simulink model "UAV_sync_unknown"  (R2018a)
settings: Solver=ode23tb  StartTime=0.0  StopTime=40
values from neighbouring files (symbols this model uses):
  Bm = [zeros(6); eye(6)]    [UAV_sync_unknown.m]    (also in UAV_sync_unknown_Node1.m = [zeros(6,6);ones(6,6)]; UAV_sync_unknown_Node2.m)
  C_rho = 1.225    [SC42120_UAV_Preconditions.m]
  D0 = [M0 0 0 0 0 0 ... (first row only)    [SC42120_UAV_Preconditions.m]
  Derivative_gain_phi = 50    [SC42120_UAV_Preconditions.m]
  Derivative_gain_psi = 50    [SC42120_UAV_Preconditions.m]
  Derivative_gain_theta = 50    [SC42120_UAV_Preconditions.m]
  Derivative_gain_x = 50    [SC42120_UAV_Preconditions.m]
  Derivative_gain_y = 50    [SC42120_UAV_Preconditions.m]
  Derivative_gain_z = 50    [SC42120_UAV_Preconditions.m]
  G = 9.80665    [SC42120_UAV_Preconditions.m]
  g0 = [0;0;-M0*G;0;0;0]    [SC42120_UAV_Preconditions.m]
  I0 = [0.02 0 -0.01 ... (first row only)    [SC42120_UAV_Preconditions.m]
  InitWind = [0;0;0]    [SC42120_UAV_Preconditions.m]
  Kp = diag(P)    [SC42120_UAV_Preconditions.m]
  Kv = diag(V)    [SC42120_UAV_Preconditions.m]
  M0 = 10    [SC42120_UAV_Preconditions.m]
  Pm = lyap(Am',-100*eye(12))    [UAV_sync_unknown_Node1.m]    (also in UAV_sync_unknown_Node2.m = lyap(Am',100*eye(12)))
  Proportional_phi = 50    [SC42120_UAV_Preconditions.m]
  Proportional_psi = 50    [SC42120_UAV_Preconditions.m]
  Proportional_theta = 50    [SC42120_UAV_Preconditions.m]
  Proportional_x = 50    [SC42120_UAV_Preconditions.m]
  Proportional_y = 50    [SC42120_UAV_Preconditions.m]
  Proportional_z = 50    [SC42120_UAV_Preconditions.m]
  S1 = eye(6)*1    [UAV_sync_unknown.m]    (also in UAV_sync_unknown_Node1.m = eye(6))
  S2 = eye(6)*1    [UAV_sync_unknown.m]    (also in UAV_sync_unknown_Node2.m)
undefined symbols (not defined in the file or in its folder): Aero, APlane, Bxl, C, Ctr, deg, DiscIntNeverNeededParam, F, Guid, Init, Light, MIL, Path, rad, s, Trim, Utility
libraries: aerolibconvert2 x37, simulink x15, dspsigops x7, shared6dof x6, aerolibasang x4, simulink_extras x3, aerolibadyn x1, aerolibtransform2 x1, aerolibwind2 x1
(part 1 of 6)
settings Model: Creator=Muhammad Ridho Rosa  LastModifiedBy=abisheknvupputur
settings SolverCC: ZeroCrossAlgorithm=Adaptive
settings CodeAppCC: StateflowObjectComments=on

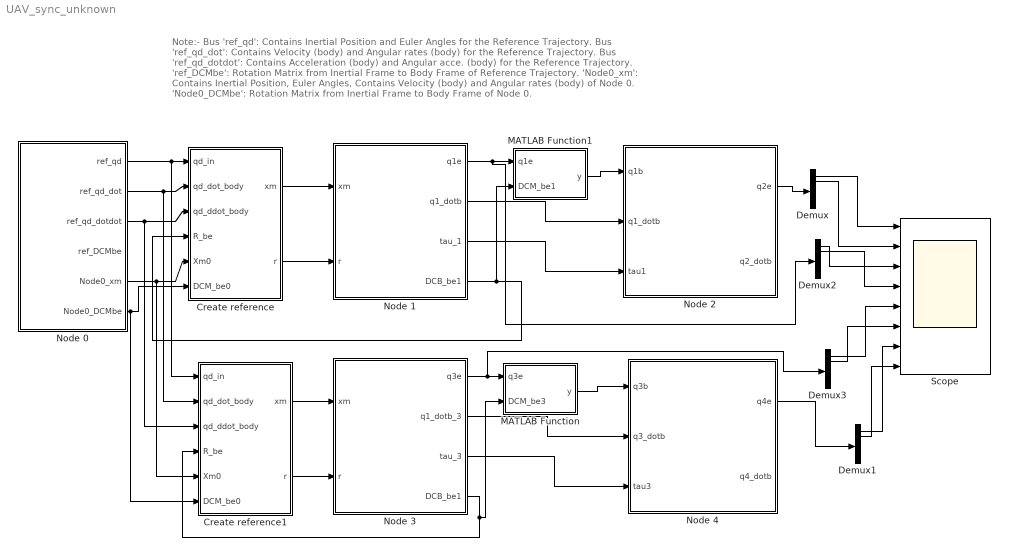
== system UAV_sync_unknown ==
  note: Note:-
      | Bus 'ref_qd': Contains Inertial Position and Euler Angles for the Reference Trajectory.
      | Bus 'ref_qd_dot': Contains Velocity (body) and Angular rates (body) for the Reference Trajectory.
      | Bus 'ref_qd_dotdot': Contains Acceleration (body) and Angular acce. (body) for the Reference Trajectory.
      | 'ref_DCMbe': Rotation Matrix from Inertial Frame to Body Frame of Reference Trajectory.
      | 'Node0_xm': Contains Inertial Position, Euler Angles, Contains Velocity (body) and Angular rates (body) of Node 0.
      | 'Node0_DCMbe': Rotation Matrix from Inertial Frame to Body Frame of Node 0.
  Create reference : Subsystem
  Create reference1 : Subsystem
  Demux{,1..3} (4 alike) : Demux  Outputs=6
  MATLAB Function : MATLAB Function  TreatAsAtomicUnit=on
  MATLAB Function1 : MATLAB Function  TreatAsAtomicUnit=on
  Node 0 : Subsystem
  Node 1 : Subsystem
  Node 2 : Subsystem
  Node 3 : Subsystem
  Node 4 : Subsystem
  Scope : Scope  NumInputPorts=8
  wires:
  Node 0/3(ref_qd_dotdot) -> Create reference1/3(qd_ddot_body), Create reference/3(qd_ddot_body)
  Node 0/2(ref_qd_dot) -> Create reference1/2(qd_dot_body), Create reference/2(qd_dot_body)
  Node 0/1(ref_qd) -> Create reference1/1(qd_in), Create reference/1(qd_in)
  Create reference/2(r) -> Node 1/2(r)
  Create reference/1(xm) -> Node 1/1(xm)
  Node 0/5(Node0_xm) -> Create reference1/5(Xm0), Create reference/5(Xm0)
  Node 0/6(Node0_DCMbe) -> Create reference1/6(DCM_be0), Create reference/6(DCM_be0)
  Create reference1/2(r) -> Node 3/2(r)
  Create reference1/1(xm) -> Node 3/1(xm)
  Node 3/4(DCB_be1) -> MATLAB Function/2(DCM_be3), Create reference1/4(R_be)
  Node 1/3(tau_1) -> Node 2/3(tau1)
  Node 1/2(q1_dotb) -> Node 2/2(q1_dotb)
  Node 3/2(q1_dotb_3) -> Node 4/2(q3_dotb)
  Node 3/3(tau_3) -> Node 4/3(tau3)
  MATLAB Function/1(y) -> Node 4/1(q3b)
  Node 3/1(q3e) -> Demux3/1, MATLAB Function/1(q3e)
  Node 1/4(DCB_be1) -> MATLAB Function1/2(DCM_be1), Create reference/4(R_be)
  Node 1/1(q1e) -> Demux2/1, MATLAB Function1/1(q1e)
  MATLAB Function1/1(y) -> Node 2/1(q1b)
  Node 2/1(q2e) -> Demux/1
  Node 4/1(q4e) -> Demux1/1
  Demux/1 -> Scope/1
  Demux/2 -> Scope/2
  Demux2/1 -> Scope/3
  Demux2/2 -> Scope/4
  Demux3/1 -> Scope/5
  Demux3/2 -> Scope/6
  Demux1/1 -> Scope/7
  Demux1/2 -> Scope/8

== system UAV_sync_unknown/Create reference ==
  qd_in : Inport
  qd_dot_body : Inport  Port=2
  qd_ddot_body : Inport  Port=3
  R_be : Inport  Port=4
  Xm0 : Inport  Port=5
  DCM_be0 : Inport  Port=6
  Demux : Demux  Outputs=2
  MATLAB Function : MATLAB Function  TreatAsAtomicUnit=on
  MATLAB Function1 : MATLAB Function  TreatAsAtomicUnit=on
  MATLAB Function2 : MATLAB Function  TreatAsAtomicUnit=on
  MATLAB Function3 : MATLAB Function  TreatAsAtomicUnit=on
  Mux : Mux  Inputs=2
  Product : Product  Multiplication=Matrix(*)
  Product1 : Product  Multiplication=Matrix(*)
  Subsystem : Subsystem
  xm : Outport
  r : Outport  Port=2
  wires:
  qd_dot_body/1 -> Subsystem/2(q_dot)
  qd_ddot_body/1 -> Subsystem/3(q_ddot)
  Subsystem/1(r) -> r/1  "r"
  Product/1 -> Subsystem/1(q)
  MATLAB Function/1(y) -> Product/1
  R_be/1 -> MATLAB Function/1(u)
  Xm0/1 -> Demux/1
  Mux/1 -> xm/1
  Product1/1 -> Mux/1
  Demux/2 -> Mux/2
  MATLAB Function1/1(y) -> Product1/1
  DCM_be0/1 -> MATLAB Function1/1(u)
  qd_in/1 -> MATLAB Function2/1(u)  "q"
  MATLAB Function2/1(y) -> Product/2
  Demux/1 -> MATLAB Function3/1(u)
  MATLAB Function3/1(y) -> Product1/2

== system UAV_sync_unknown/Create reference1 ==
  qd_in : Inport
  qd_dot_body : Inport  Port=2
  qd_ddot_body : Inport  Port=3
  R_be : Inport  Port=4
  Xm0 : Inport  Port=5
  DCM_be0 : Inport  Port=6
  Demux : Demux  Outputs=2
  MATLAB Function : MATLAB Function  TreatAsAtomicUnit=on
  MATLAB Function1 : MATLAB Function  TreatAsAtomicUnit=on
  MATLAB Function2 : MATLAB Function  TreatAsAtomicUnit=on
  MATLAB Function3 : MATLAB Function  TreatAsAtomicUnit=on
  Mux : Mux  Inputs=2
  Product : Product  Multiplication=Matrix(*)
  Product1 : Product  Multiplication=Matrix(*)
  Subsystem : Subsystem
  xm : Outport
  r : Outport  Port=2
  wires:
  qd_dot_body/1 -> Subsystem/2(q_dot)
  qd_ddot_body/1 -> Subsystem/3(q_ddot)
  Subsystem/1(r) -> r/1  "r"
  Product/1 -> Subsystem/1(q)
  MATLAB Function/1(y) -> Product/1
  R_be/1 -> MATLAB Function/1(u)
  Xm0/1 -> Demux/1
  Mux/1 -> xm/1
  Product1/1 -> Mux/1
  Demux/2 -> Mux/2
  MATLAB Function1/1(y) -> Product1/1
  DCM_be0/1 -> MATLAB Function1/1(u)
  qd_in/1 -> MATLAB Function2/1(u)  "q"
  MATLAB Function2/1(y) -> Product/2
  Demux/1 -> MATLAB Function3/1(u)
  MATLAB Function3/1(y) -> Product1/2

== system UAV_sync_unknown/Node 0 ==
  Bus Creator : BusCreator  Inputs=2
  Bus Creator1 : BusCreator  Inputs=2
  Bus Creator2 : BusCreator  Inputs=2
  Bus Creator3 : BusCreator  Inputs=4
  Bus Selector : BusSelector  OutputSignals=PlantData.Position (inertial),PlantData.Euler angles (rad),PlantData.Velocity (body),PlantData.Angular rates (body) (rad/s),PlantData.Accelerations (body/body),PlantData.Angular accelerations (body/body),PlantData.From inertial to body matrix
  Bus Selector1 : BusSelector  OutputSignals=Position (inertial),Euler angles (rad),Velocity (body),Angular rates (body),MatrixTransformation(Inertial-Body)
  Node 0 : Subsystem
  VF Approach : Subsystem
  ref_qd : Outport
  ref_qd_dot : Outport  Port=2
  ref_qd_dotdot : Outport  Port=3
  ref_DCMbe : Outport  Port=4
  Node0_xm : Outport  Port=5
  Node0_DCMbe : Outport  Port=6
  wires:
  VF Approach/1(VF_System_Parameters) -> Node 0/1(VF_System_Parameters)
  VF Approach/2(PlantData) -> Bus Selector/1
  Bus Selector/1 -> Bus Creator/1  "<Position (inertial)>"
  Bus Selector/2 -> Bus Creator/2  "<Euler angles (rad)>"
  Bus Creator/1 -> ref_qd/1
  Bus Selector/4 -> Bus Creator1/2  "<Angular rates (body) (rad/s)>"
  Bus Selector/3 -> Bus Creator1/1  "<Velocity (body)>"
  Bus Creator1/1 -> ref_qd_dot/1
  Bus Selector/6 -> Bus Creator2/2  "<Angular accelerations (body/body)>"
  Bus Selector/5 -> Bus Creator2/1  "<Accelerations (body/body)>"
  Bus Creator2/1 -> ref_qd_dotdot/1
  Bus Selector/7 -> ref_DCMbe/1  "<From inertial to body matrix>"
  Node 0/1(Node0_Data) -> Bus Selector1/1
  Bus Selector1/1 -> Bus Creator3/1  "<Position (inertial)>"
  Bus Selector1/3 -> Bus Creator3/3  "<Velocity (body)>"
  Bus Selector1/4 -> Bus Creator3/4  "<Angular rates (body)>"
  Bus Creator3/1 -> Node0_xm/1
  Bus Selector1/5 -> Node0_DCMbe/1  "<MatrixTransformation(Inertial-Body)>"
  Bus Selector1/2 -> Bus Creator3/2  "<Euler angles (rad)>"

== system UAV_sync_unknown/Node 1 ==
  note: Error
  note: q1_dotb
  xm : Inport
  r : Inport  Port=2
  Demux : Demux  Outputs=2
  NODE1_6DOF : Subsystem
  Reshape1 : Reshape  OutputDimensionality=Column vector (2-D)
  Reshape7 : Reshape  OutputDimensionality=Row vector (2-D)
  Scope : Scope
  Subsystem : Subsystem
  Subsystem1 : Subsystem
  Subsystem2 : Subsystem
  Subsystem3 : Subsystem
  Sum1 : Sum  Inputs=|-+
  Sum2 : Sum
  Terminator1 : Terminator
  Terminator2 : Terminator
  Vector Concatenate4 : Concatenate
  q1e : Outport
  q1_dotb : Outport  Port=2
  tau_1 : Outport  Port=3
  DCB_be1 : Outport  Port=4
  wires:
  Sum1/1 -> Reshape1/1, Scope/1
  Sum2/1 -> tau_1/1, Demux/1
  Vector Concatenate4/1 -> Sum1/2  "q1"
  NODE1_6DOF/4(q1_dotb) -> Subsystem3/3(q1_dot), Subsystem/2(q1_dot_b), q1_dotb/1, Vector Concatenate4/2
  Demux/1 -> NODE1_6DOF/1("F_{xyz}")
  Demux/2 -> NODE1_6DOF/2("M_{xyz}")
  NODE1_6DOF/2(q1_dote) -> Terminator1/1
  NODE1_6DOF/6(DCMbe1) -> DCB_be1/1
  NODE1_6DOF/3(q1) -> Subsystem3/2(q1), Vector Concatenate4/1
  xm/1 -> Reshape7/1
  Reshape7/1 -> Sum1/1
  Subsystem/1(C*q1) -> Sum2/2
  Subsystem1/1(D(-Kpq-Kvq_dot+r)) -> Sum2/1
  Subsystem2/1(-S1.Bm'.P.e) -> Subsystem/1(-S1.Bm'.P.e), Subsystem1/2(-S1.Bm'.P.e)
  Reshape1/1 -> Subsystem2/1(e)
  r/1 -> Subsystem3/1(r)
  Subsystem3/1((-Kpq-Kvq_dot+r)) -> Subsystem1/1((-Kpq-Kvq_dot+r))
  NODE1_6DOF/1(q1e) -> q1e/1
  NODE1_6DOF/5(Xe1) -> Terminator2/1

== system UAV_sync_unknown/Node 2 ==
  note: tau2
  note: D2_D1_C1*q1dot
  note: q1dot
  note: D2_D1*tau1
  note: Xi_D2_D1
  note: Xi_D2_D1dot
  note: D2*()
  note: Theta_D2
  note: Theta_D2dot
  note: Kv
  note: Kp
  note: pqr
  note: C2*q2_
      | dot
  note: Theta_C2
  note: Theta_C2dot
  note: e_21
  q1b : Inport
  q1_dotb : Inport  Port=2
  tau1 : Inport  Port=3
  Constant : Constant  Value=-S2*Bm'
  Constant1 : Constant  Value=S2*Bm'
  Constant2 : Constant  Value=-S2*Bm'
  Constant3 : Constant  Value=S2*Bm'
  Demux2 : Demux  Outputs=2
  Gain{,1,4..5} (4 alike) : Gain  Gain=Pm  Multiplication=Matrix(u*K)
  Gain2 : Gain  Gain=Kp  Multiplication=Matrix(K*u)
  Gain3 : Gain  Gain=Kv  Multiplication=Matrix(K*u)
  Integrator{,1..3} (4 alike) : Integrator
  Math Function{,1..4} (5 alike) : Math  Operator=transpose  SaturateOnIntegerOverflow=on
  Node2_6DOF : Subsystem
  Product{1,4,7..8} (4 alike) : Product  Inputs=3  Multiplication=Matrix(*)
  Product2 : Product  Multiplication=Matrix(*)
  Product3 : Product  Inputs=4  Multiplication=Matrix(*)
  Product5 : Product  Multiplication=Matrix(*)
  Product6 : Product  Inputs=4  Multiplication=Matrix(*)
  Reshape1 : Reshape  OutputDimensionality=Column vector (2-D)
  Reshape2 : Reshape  OutputDimensionality=Row vector (2-D)
  Reshape5 : Reshape  OutputDimensionality=Row vector (2-D)
  Scope : Scope
  Sum : Sum  Inputs=|+-
  Sum1 : Sum  Inputs=|+-
  Sum2 : Sum  Inputs=|++
  Sum3 : Sum  Inputs=|-++-
  Terminator : Terminator
  Terminator1 : Terminator
  Terminator2 : Terminator
  Vector Concatenate4 : Concatenate
  "Xi_C " : MATLAB Function  TreatAsAtomicUnit=on
  "Xi_D_D_C " : MATLAB Function  TreatAsAtomicUnit=on
  q2e : Outport
  q2_dotb : Outport  Port=2
  wires:
  Node2_6DOF/1(q2e) -> q2e/1
  Node2_6DOF/3(q2b) -> Sum/1
  q1b/1 -> Sum/2
  Sum1/1 -> Gain3/1, Vector Concatenate4/2
  Node2_6DOF/4(q2_dotb) -> q2_dotb/1, Product7/3, Sum1/1, Reshape2/1
  Gain/1 -> Product3/1
  Constant/1 -> Gain/1
  Vector Concatenate4/1 -> Scope/1, Reshape1/1
  Reshape1/1 -> Product1/2, Product4/2, Product6/2, Product3/2
  Reshape2/1 -> Product3/3
  "Xi_C "/1(y) -> Math Function/1, Product3/4
  Product3/1 -> Integrator/1
  Integrator/1 -> Product7/1
  Math Function/1 -> Product7/2
  Constant1/1 -> Gain1/1
  Gain1/1 -> Product1/1
  Sum/1 -> Gain2/1, Vector Concatenate4/1
  Gain2/1 -> Sum2/1
  Gain3/1 -> Sum2/2
  Sum2/1 -> Math Function2/1
  Product1/1 -> Integrator1/1
  Integrator1/1 -> Product2/1
  Constant2/1 -> Gain4/1
  Gain4/1 -> Product4/1
  tau1/1 -> Reshape5/1, Product5/2
  Product4/1 -> Integrator2/1
  Integrator2/1 -> Product5/1
  Constant3/1 -> Gain5/1
  Gain5/1 -> Product6/1
  Math Function4/1 -> Product6/3
  Reshape5/1 -> Product4/3
  "Xi_D_D_C "/1(y) -> Product8/2, Math Function1/1
  Math Function1/1 -> Product6/4
  Product6/1 -> Integrator3/1
  Integrator3/1 -> Product8/1
  q1_dotb/1 -> Product8/3, Math Function4/1, Sum1/2
  Product2/1 -> Sum3/1
  Product7/1 -> Sum3/2
  Product5/1 -> Sum3/3
  Sum3/1 -> Demux2/1
  Demux2/1 -> Node2_6DOF/1("F_{xyz}")
  Demux2/2 -> Node2_6DOF/2("M_{xyz}")
  Math Function2/1 -> Math Function3/1, Product1/3
  Math Function3/1 -> Product2/2
  Product8/1 -> Sum3/4
  Node2_6DOF/7(omega_b2) -> "Xi_D_D_C "/1(u), "Xi_C "/1(u)
  Node2_6DOF/5(Xe2) -> Terminator/1
  Node2_6DOF/6(DCMbe2) -> Terminator1/1
  Node2_6DOF/2(q2_dote) -> Terminator2/1

== system UAV_sync_unknown/Node 3 ==
  note: Error
  note: q1_dotb
  xm : Inport
  r : Inport  Port=2
  Demux : Demux  Outputs=2
  NODE1_6DOF : Subsystem
  Reshape1 : Reshape  OutputDimensionality=Column vector (2-D)
  Reshape7 : Reshape  OutputDimensionality=Row vector (2-D)
  Scope : Scope
  Subsystem : Subsystem
  Subsystem1 : Subsystem
  Subsystem2 : Subsystem
  Subsystem3 : Subsystem
  Sum1 : Sum  Inputs=|-+
  Sum2 : Sum
  Terminator1 : Terminator
  Terminator2 : Terminator
  Vector Concatenate4 : Concatenate
  q3e : Outport
  q1_dotb_3 : Outport  Port=2
  tau_3 : Outport  Port=3
  DCB_be1 : Outport  Port=4
  wires:
  Sum1/1 -> Reshape1/1, Scope/1
  Sum2/1 -> tau_3/1, Demux/1
  Vector Concatenate4/1 -> Sum1/2  "q1"
  NODE1_6DOF/4(q1_dotb) -> Subsystem3/3(q1_dot), Subsystem/2(q1_dot_b), q1_dotb_3/1, Vector Concatenate4/2
  Demux/1 -> NODE1_6DOF/1("F_{xyz}")
  Demux/2 -> NODE1_6DOF/2("M_{xyz}")
  NODE1_6DOF/2(q1_dote) -> Terminator1/1
  NODE1_6DOF/6(DCMbe1) -> DCB_be1/1
  NODE1_6DOF/3(q1) -> Subsystem3/2(q1), Vector Concatenate4/1
  xm/1 -> Reshape7/1
  Reshape7/1 -> Sum1/1
  Subsystem/1(C*q1) -> Sum2/2
  Subsystem1/1(D(-Kpq-Kvq_dot+r)) -> Sum2/1
  Subsystem2/1(-S1.Bm'.P.e) -> Subsystem/1(-S1.Bm'.P.e), Subsystem1/2(-S1.Bm'.P.e)
  Reshape1/1 -> Subsystem2/1(e)
  r/1 -> Subsystem3/1(r)
  Subsystem3/1((-Kpq-Kvq_dot+r)) -> Subsystem1/1((-Kpq-Kvq_dot+r))
  NODE1_6DOF/1(q1e) -> q3e/1
  NODE1_6DOF/5(Xe1) -> Terminator2/1

== system UAV_sync_unknown/Node 4 ==
  note: tau4
  note: D2_D1_C1*q1dot
  note: q1dot
  note: D2_D1*tau1
  note: Xi_D2_D1
  note: Xi_D2_D1dot
  note: D2*()
  note: Theta_D2
  note: Theta_D2dot
  note: Kv
  note: Kp
  note: pqr
  note: C2*q2_
      | dot
  note: Theta_C2
  note: Theta_C2dot
  note: e_34
  q3b : Inport
  q3_dotb : Inport  Port=2
  tau3 : Inport  Port=3
  Constant : Constant  Value=-S2*Bm'
  Constant1 : Constant  Value=S2*Bm'
  Constant2 : Constant  Value=-S2*Bm'
  Constant3 : Constant  Value=S2*Bm'
  Demux2 : Demux  Outputs=2
  Gain{,1,4..5} (4 alike) : Gain  Gain=Pm  Multiplication=Matrix(u*K)
  Gain2 : Gain  Gain=Kp  Multiplication=Matrix(K*u)
  Gain3 : Gain  Gain=Kv  Multiplication=Matrix(K*u)
  Integrator{,1..3} (4 alike) : Integrator
  Math Function{,1..4} (5 alike) : Math  Operator=transpose  SaturateOnIntegerOverflow=on
  Node2_6DOF : Subsystem
  Product{1,4,7..8} (4 alike) : Product  Inputs=3  Multiplication=Matrix(*)
  Product2 : Product  Multiplication=Matrix(*)
  Product3 : Product  Inputs=4  Multiplication=Matrix(*)
  Product5 : Product  Multiplication=Matrix(*)
  Product6 : Product  Inputs=4  Multiplication=Matrix(*)
  Reshape1 : Reshape  OutputDimensionality=Column vector (2-D)
  Reshape2 : Reshape  OutputDimensionality=Row vector (2-D)
  Reshape5 : Reshape  OutputDimensionality=Row vector (2-D)
  Scope : Scope
  Sum : Sum  Inputs=|+-
  Sum1 : Sum  Inputs=|+-
  Sum2 : Sum  Inputs=|++
  Sum3 : Sum  Inputs=|-++-
  Terminator : Terminator
  Terminator1 : Terminator
  Terminator2 : Terminator
  Vector Concatenate4 : Concatenate
  "Xi_C " : MATLAB Function  TreatAsAtomicUnit=on
  "Xi_D_D_C " : MATLAB Function  TreatAsAtomicUnit=on
  q4e : Outport
  q4_dotb : Outport  Port=2
  wires:
  Node2_6DOF/1(q4e) -> q4e/1
  Node2_6DOF/3(q4b) -> Sum/1
  q3b/1 -> Sum/2
  Sum1/1 -> Gain3/1, Vector Concatenate4/2
  Node2_6DOF/4(q4_dotb) -> q4_dotb/1, Product7/3, Sum1/1, Reshape2/1
  Gain/1 -> Product3/1
  Constant/1 -> Gain/1
  Vector Concatenate4/1 -> Scope/1, Reshape1/1
  Reshape1/1 -> Product1/2, Product4/2, Product6/2, Product3/2
  Reshape2/1 -> Product3/3
  "Xi_C "/1(y) -> Math Function/1, Product3/4
  Product3/1 -> Integrator/1
  Integrator/1 -> Product7/1
  Math Function/1 -> Product7/2
  Constant1/1 -> Gain1/1
  Gain1/1 -> Product1/1
  Sum/1 -> Gain2/1, Vector Concatenate4/1
  Gain2/1 -> Sum2/1
  Gain3/1 -> Sum2/2
  Sum2/1 -> Math Function2/1
  Product1/1 -> Integrator1/1
  Integrator1/1 -> Product2/1
  Constant2/1 -> Gain4/1
  Gain4/1 -> Product4/1
  tau3/1 -> Reshape5/1, Product5/2
  Product4/1 -> Integrator2/1
  Integrator2/1 -> Product5/1
  Constant3/1 -> Gain5/1
  Gain5/1 -> Product6/1
  Math Function4/1 -> Product6/3
  Reshape5/1 -> Product4/3
  "Xi_D_D_C "/1(y) -> Product8/2, Math Function1/1
  Math Function1/1 -> Product6/4
  Product6/1 -> Integrator3/1
  Integrator3/1 -> Product8/1
  q3_dotb/1 -> Product8/3, Math Function4/1, Sum1/2
  Product2/1 -> Sum3/1
  Product7/1 -> Sum3/2
  Product5/1 -> Sum3/3
  Sum3/1 -> Demux2/1
  Demux2/1 -> Node2_6DOF/1("F_{xyz}")
  Demux2/2 -> Node2_6DOF/2("M_{xyz}")
  Math Function2/1 -> Math Function3/1, Product1/3
  Math Function3/1 -> Product2/2
  Product8/1 -> Sum3/4
  Node2_6DOF/7(omega_b4) -> "Xi_D_D_C "/1(u), "Xi_C "/1(u)
  Node2_6DOF/5(Xe4) -> Terminator/1
  Node2_6DOF/6(DCMbe4) -> Terminator1/1
  Node2_6DOF/2(q4_dote) -> Terminator2/1

== system UAV_sync_unknown/Create reference/Subsystem ==
  q : Inport
  q_dot : Inport  Port=2
  q_ddot : Inport  Port=3
  Gain : Gain  Gain=Kv  Multiplication=Matrix(K*u)
  Gain1 : Gain  Gain=Kp  Multiplication=Matrix(K*u)
  Sum : Sum  Inputs=+++
  r : Outport
  wires:
  Gain1/1 -> Sum/1
  q/1 -> Gain1/1
  q_dot/1 -> Gain/1
  q_ddot/1 -> Sum/3
  Sum/1 -> r/1  "r"
  Gain/1 -> Sum/2

== system UAV_sync_unknown/Create reference1/Subsystem ==
  q : Inport
  q_dot : Inport  Port=2
  q_ddot : Inport  Port=3
  Gain : Gain  Gain=Kv  Multiplication=Matrix(K*u)
  Gain1 : Gain  Gain=Kp  Multiplication=Matrix(K*u)
  Sum : Sum  Inputs=+++
  r : Outport
  wires:
  Gain1/1 -> Sum/1
  q/1 -> Gain1/1
  q_dot/1 -> Gain/1
  q_ddot/1 -> Sum/3
  Sum/1 -> r/1  "r"
  Gain/1 -> Sum/2

== system UAV_sync_unknown/Node 0/Node 0 ==
  note: Inverse Dynamics
  VF_System_Parameters : Inport
  6DOF (Euler Angles) : shared6dof/6DOF (Euler Angles)  units=Metric (MKS)  mtype=Fixed  rep=Euler Angles  xme_0=init_pos0  Vm_0=init_vel0  eul_0=init_eul0  pm_0=init_ang0  mass_0=M0  mass_e=0.5  mass_f=2.0  inertia=I0  inertia_e=eye(3)  inertia_f=2*eye(3)  k_quat=1.0  vre_flag=on  abi_flag=off  aMode=aMode
      settings: SourceProductBaseCode=AE
  ALL_DATA2 : Goto  Commented=on  GotoTag=DERIVED_DATA
  Add : Sum
  Bus Creator : BusCreator  Inputs=10
  Constant8 : Constant  Value=M0*G
  Demux5 : Demux  Outputs=6
  Derived Data : Subsystem
  Gain : Gain  Gain=[1 1 -1]
  Inverse Dynamics Control : Subsystem
  Mux8 : Mux  Inputs=3
  Mux9 : Mux  Inputs=3
  Product : Product  Multiplication=Matrix(*)
  Subsystem : Subsystem
  Wind : Subsystem
  tau : Sum  Inputs=+++
  Node0_Data : Outport
  wires:
  Gain/1 -> Product/2, Bus Creator/3  "xyh"
  6DOF (Euler Angles)/1 -> Bus Creator/1  "Velocity (inertial)"
  Mux8/1 -> 6DOF (Euler Angles)/1
  6DOF (Euler Angles)/3 -> Bus Creator/4  "Euler angles (rad)"
  Bus Creator/1 -> [AIRCRAFT_DATA]
  6DOF (Euler Angles)/6 -> Bus Creator/7  "Angular rates (body)"
  6DOF (Euler Angles)/8 -> Bus Creator/9  "Acceleration (Body)"
  Mux9/1 -> 6DOF (Euler Angles)/2
  6DOF (Euler Angles)/7 -> Bus Creator/8  "Angular accelerations (body)"
  6DOF (Euler Angles)/5 -> Bus Creator/6  "Velocity (body)"
  6DOF (Euler Angles)/2 -> Gain/1, Bus Creator/2  "Position (inertial)"
  6DOF (Euler Angles)/4 -> Product/1, Bus Creator/5  "MatrixTransformation(Inertial-Body)"
  tau/1 -> Demux5/1
  Demux5/2 -> Mux8/2
  Demux5/4 -> Mux9/1
  Demux5/5 -> Mux9/2
  Demux5/6 -> Mux9/3
  [WIND_DATA] -> Derived Data/1(In1)
  [AIRCRAFT_DATA] -> Derived Data/2(In2)
  Derived Data/1(Derived_Condition) -> ALL_DATA2/1
  [AIRCRAFT_DATA] -> Wind/1(In1)
  Wind/1(Out1) -> [WIND_DATA]
  Inverse Dynamics Control/1(D_qddot) -> tau/1
  Inverse Dynamics Control/2(C_qdot) -> tau/2
  Inverse Dynamics Control/3(g(q)) -> tau/3
  Constant8/1 -> Add/2
  Demux5/3 -> Add/1
  Add/1 -> Mux8/3
  Demux5/1 -> Mux8/1
  [AIRCRAFT_DATA] -> Inverse Dynamics Control/2(Aircraft Data), Node0_Data/1
  VF_System_Parameters/1 -> Subsystem/1(VF_System_Parameters)
  Subsystem/1(References) -> Inverse Dynamics Control/1(References)
  Product/1 -> Bus Creator/10  "xyh_body"

== system UAV_sync_unknown/Node 0/VF Approach ==
  note: Created by: Stefano Farì
      | Last edit: Mar 2018
  note: Fixed-wing UAV Simulator
  note: Ground Hit
  note: Wind
  note: To workspace
  note: MAIN
  AUTOPILOT : Subsystem
  BIXLER DYNAMICS : Subsystem
  Bus Selector3 : BusSelector  OutputSignals=PlantData.xyh_body,PlantData.Euler angles (rad),PlantData.Velocity (body),PlantData.Angular rates (body) (rad/s),PlantData.Accelerations (body/body),PlantData.Angular accelerations (body/body)
  ENVIRONMENT : Subsystem
  GROUND HIT : Subsystem
  MANUAL INPUTS : Subsystem
  Mux : Mux  Inputs=6
  PATH FOLLOWING : Subsystem
  PATH MANAGER : Subsystem
  TO WORKSPACE : Subsystem
  VF_System_Parameters : Outport
  PlantData : Outport  Port=2
  wires:
  MANUAL INPUTS/2(EnvData.) -> BIXLER DYNAMICS/2(EnvData)
  [PlantData] -> PATH MANAGER/1(PlantData)
  MANUAL INPUTS/4(VF.) -> BIXLER DYNAMICS/4(VF)
  [VF] -> TO WORKSPACE/4(VF)
  MANUAL INPUTS/3(GuidData.) -> BIXLER DYNAMICS/3(GuidData)
  [EnvData] -> PATH MANAGER/3(EnvData)
  [PlantData] -> PlantData/1, Bus Selector3/1
  BIXLER DYNAMICS/4(GuidData.) -> [GuidData]
  MANUAL INPUTS/1(CtrBus.) -> BIXLER DYNAMICS/1(ControlActions)
  AUTOPILOT/3(VF.) -> MANUAL INPUTS/3(VF)
  PATH MANAGER/2(DerCond.) -> PATH FOLLOWING/2(DerCond)
  PATH FOLLOWING/1("PlantData. ") -> AUTOPILOT/1(PlantData)
  AUTOPILOT/4(GuidData.) -> MANUAL INPUTS/4(GuidData)
  [GuidData] -> TO WORKSPACE/5(GuidData)
  [DerCond] -> TO WORKSPACE/2(DerCond)
  PATH FOLLOWING/5(GuidData.) -> AUTOPILOT/5(GuidData)
  BIXLER DYNAMICS/5(VF.) -> [VF]
  PATH FOLLOWING/2("DerCond. ") -> AUTOPILOT/2(DerCond)
  BIXLER DYNAMICS/1(PlantData.) -> [PlantData]
  [PlantData] -> GROUND HIT/1(PlantData)
  [PlantData] -> ENVIRONMENT/1(PlantData)
  BIXLER DYNAMICS/3(ControlBus.) -> [ControlBus]
  AUTOPILOT/2(EnvData.) -> MANUAL INPUTS/2(EnvData)
  PATH MANAGER/1(Plantdata.) -> PATH FOLLOWING/1(PlantData)
  PATH MANAGER/4(GuidData.) -> PATH FOLLOWING/4(GuidData)
  ENVIRONMENT/1(EnvData) -> [EnvData]
  PATH FOLLOWING/4(VF.) -> AUTOPILOT/4(VF)
  Bus Selector3/4 -> Mux/4  "<Angular rates (body) (rad/s)>"
  PATH MANAGER/3(EnvData.) -> PATH FOLLOWING/3(EnvData)
  [PlantData] -> TO WORKSPACE/1(PlantData)
  [DerCond] -> PATH MANAGER/2(DerCond)
  BIXLER DYNAMICS/2(DerCond.) -> [DerCond]
  [EnvData] -> TO WORKSPACE/6(EnvData)
  [ControlBus] -> TO WORKSPACE/3(ControlBus)
  AUTOPILOT/1(CtrBus.) -> MANUAL INPUTS/1(CtrBus)
  PATH FOLLOWING/3(EnvData.) -> AUTOPILOT/3(EnvData)
  Mux/1 -> VF_System_Parameters/1
  Bus Selector3/1 -> Mux/1  "<xyh_body>"
  Bus Selector3/2 -> Mux/2  "<Euler angles (rad)>"
  Bus Selector3/3 -> Mux/3  "<Velocity (body)>"
  Bus Selector3/5 -> Mux/5  "<Accelerations (body/body)>"
  Bus Selector3/6 -> Mux/6  "<Angular accelerations (body/body)>"

== system UAV_sync_unknown/Node 1/NODE1_6DOF ==
  "F_{xyz}" : Inport
  "M_{xyz}" : Inport  Port=2
  6DOF (Euler Angles) Node 1 : shared6dof/6DOF (Euler Angles)  units=Metric (MKS)  mtype=Fixed  rep=Euler Angles  xme_0=init_pos1  Vm_0=init_vel1  eul_0=init_eul1  pm_0=init_ang1  mass_0=M1  mass_e=0.5  mass_f=2.0  inertia=I1  inertia_e=eye(3)  inertia_f=2*eye(3)  k_quat=1.0  vre_flag=on  abi_flag=on  aMode=aMode
      settings: SourceProductBaseCode=AE
  Product : Product  Multiplication=Matrix(*)
  Terminator1 : Terminator
  Terminator2 : Terminator
  Terminator3 : Terminator
  Vector Concatenate{,1..3} (4 alike) : Concatenate
  q1e : Outport
  q1_dote : Outport  Port=2
  q1 : Outport  Port=3
  q1_dotb : Outport  Port=4
  Xe1 : Outport  Port=5
  DCMbe1 : Outport  Port=6
  wires:
  Vector Concatenate2/1 -> q1e/1  "q1"
  Vector Concatenate3/1 -> q1_dote/1  "q1_dot"
  6DOF (Euler Angles) Node 1/7 -> Terminator1/1
  6DOF (Euler Angles) Node 1/6 -> Vector Concatenate3/2, Vector Concatenate1/2
  6DOF (Euler Angles) Node 1/8 -> Terminator2/1
  6DOF (Euler Angles) Node 1/5 -> Vector Concatenate1/1
  Product/1 -> Vector Concatenate/1
  Vector Concatenate1/1 -> q1_dotb/1  "q1_dot"
  6DOF (Euler Angles) Node 1/1 -> Vector Concatenate3/1
  "F_{xyz}"/1 -> 6DOF (Euler Angles) Node 1/1
  6DOF (Euler Angles) Node 1/3 -> Vector Concatenate2/2, Vector Concatenate/2
  "M_{xyz}"/1 -> 6DOF (Euler Angles) Node 1/2
  Vector Concatenate/1 -> q1/1  "q1"
  6DOF (Euler Angles) Node 1/2 -> Xe1/1, Product/2, Vector Concatenate2/1
  6DOF (Euler Angles) Node 1/4 -> DCMbe1/1, Product/1
  6DOF (Euler Angles) Node 1/9 -> Terminator3/1

== system UAV_sync_unknown/Node 1/Subsystem ==
  note: C_Part
  note: theta_C
  note: q1_dotb
  note: -S1.Bm'.P.e.q_dot
  note: -S1.Bm'.P.e.q_dot.Xi_C
  -S1.Bm'.P.e : Inport
  q1_dot_b : Inport  Port=2
  Integrator1 : Integrator
  Product{3..4,6..7} (4 alike) : Product  Multiplication=Matrix(*)
  Reshape3 : Reshape  OutputDimensionality=Row vector (2-D)
  Reshape5 : Reshape  OutputDimensionality=Column vector (2-D)
  To Workspace1 : ToWorkspace  Commented=on  VariableName=Theta_C  SaveFormat=Structure With Time  SampleTime=-1
      settings: Decimation=2
  Transpose1 : Math  Operator=transpose  SaturateOnIntegerOverflow=on
  "Xi_C " : MATLAB Function  TreatAsAtomicUnit=on
  C*q1 : Outport
  wires:
  Product3/1 -> Product4/1
  Transpose1/1 -> Product6/2
  Reshape5/1 -> C*q1/1
  Reshape3/1 -> Product3/2
  -S1.Bm'.P.e/1 -> Product3/1
  Product4/1 -> Integrator1/1
  "Xi_C "/1(y) -> Transpose1/1, Product4/2
  Product6/1 -> Product7/1
  q1_dot_b/1 -> Reshape3/1, Product7/2, "Xi_C "/1(u)
  Product7/1 -> Reshape5/1
  Integrator1/1 -> To Workspace1/1, Product6/1

== system UAV_sync_unknown/Node 1/Subsystem1 ==
  note: D_Part
  note: theta_D
  note: Xi_D=> eye(6)
  note: -S1.Bm'.P.e.()
  (-Kpq-Kvq_dot+r) : Inport
  -S1.Bm'.P.e : Inport  Port=2
  Integrator : Integrator
  Product2 : Product  Multiplication=Matrix(*)
  Product5 : Product  Multiplication=Matrix(*)
  Reshape2 : Reshape  OutputDimensionality=Row vector (2-D)
  Reshape4 : Reshape  OutputDimensionality=Column vector (2-D)
  Reshape6 : Reshape  OutputDimensionality=Column vector (2-D)
  To Workspace : ToWorkspace  Commented=on  VariableName=Theta_D  SaveFormat=Structure With Time  SampleTime=-1
      settings: Decimation=2
  D(-Kpq-Kvq_dot+r) : Outport
  wires:
  Reshape6/1 -> D(-Kpq-Kvq_dot+r)/1
  -S1.Bm'.P.e/1 -> Product2/1
  Reshape4/1 -> Product5/2
  Product2/1 -> Integrator/1
  Integrator/1 -> Product5/1, To Workspace/1
  (-Kpq-Kvq_dot+r)/1 -> Reshape2/1
  Reshape2/1 -> Reshape4/1, Product2/2
  Product5/1 -> Reshape6/1

== system UAV_sync_unknown/Node 1/Subsystem2 ==
  note: -S1.Bm'.P.e
  e : Inport
  Constant : Constant  Value=-100*S1*Bm'
  P : Gain  Gain=Pm  Multiplication=Matrix(u*K)
  Product1 : Product  Multiplication=Matrix(*)
  -S1.Bm'.P.e : Outport
  wires:
  Product1/1 -> -S1.Bm'.P.e/1
  e/1 -> Product1/2
  P/1 -> Product1/1
  Constant/1 -> P/1

== system UAV_sync_unknown/Node 1/Subsystem3 ==
  r : Inport
  q1 : Inport  Port=2
  q1_dot : Inport  Port=3
  Gain1 : Gain  Gain=Kv  Multiplication=Matrix(K*u)
  Gain2 : Gain  Gain=Kp  Multiplication=Matrix(K*u)
  Sum : Sum  Inputs=-+-
  (-Kpq-Kvq_dot+r) : Outport
  wires:
  Sum/1 -> (-Kpq-Kvq_dot+r)/1
  r/1 -> Sum/2
  Gain2/1 -> Sum/1
  q1_dot/1 -> Gain1/1
  Gain1/1 -> Sum/3
  q1/1 -> Gain2/1

== system UAV_sync_unknown/Node 2/Node2_6DOF ==
  "F_{xyz}" : Inport
  "M_{xyz}" : Inport  Port=2
  6DOF (Euler Angles) Node 2 : shared6dof/6DOF (Euler Angles)  units=Metric (MKS)  mtype=Fixed  rep=Euler Angles  xme_0=init_pos2  Vm_0=init_vel2  eul_0=init_eul2  pm_0=init_ang2  mass_0=M2  mass_e=0.5  mass_f=2.0  inertia=I1  inertia_e=eye(3)  inertia_f=2*eye(3)  k_quat=1.0  vre_flag=on  abi_flag=on  aMode=aMode
      settings: SourceProductBaseCode=AE
  Product : Product  Multiplication=Matrix(*)
  Terminator1 : Terminator
  Terminator2 : Terminator
  Terminator3 : Terminator
  Vector Concatenate{,1..3} (4 alike) : Concatenate
  q2e : Outport
  q2_dote : Outport  Port=2
  q2b : Outport  Port=3
  q2_dotb : Outport  Port=4
  Xe2 : Outport  Port=5
  DCMbe2 : Outport  Port=6
  omega_b2 : Outport  Port=7
  wires:
  "M_{xyz}"/1 -> 6DOF (Euler Angles) Node 2/2
  Vector Concatenate1/1 -> q2_dotb/1  "q2_dot"
  "F_{xyz}"/1 -> 6DOF (Euler Angles) Node 2/1
  6DOF (Euler Angles) Node 2/8 -> Terminator2/1
  Vector Concatenate/1 -> q2b/1  "q2"
  6DOF (Euler Angles) Node 2/9 -> Terminator3/1
  Product/1 -> Vector Concatenate/1
  Vector Concatenate2/1 -> q2e/1  "q2"
  Vector Concatenate3/1 -> q2_dote/1  "q2_dot"
  6DOF (Euler Angles) Node 2/7 -> Terminator1/1
  6DOF (Euler Angles) Node 2/1 -> Vector Concatenate3/1
  6DOF (Euler Angles) Node 2/2 -> Vector Concatenate2/1, Xe2/1, Product/2
  6DOF (Euler Angles) Node 2/4 -> DCMbe2/1, Product/1
  6DOF (Euler Angles) Node 2/3 -> Vector Concatenate2/2, Vector Concatenate/2
  6DOF (Euler Angles) Node 2/6 -> Vector Concatenate3/2, omega_b2/1, Vector Concatenate1/2
  6DOF (Euler Angles) Node 2/5 -> Vector Concatenate1/1

== system UAV_sync_unknown/Node 3/NODE1_6DOF ==
  "F_{xyz}" : Inport
  "M_{xyz}" : Inport  Port=2
  6DOF (Euler Angles) Node 1 : shared6dof/6DOF (Euler Angles)  units=Metric (MKS)  mtype=Fixed  rep=Euler Angles  xme_0=init_pos3  Vm_0=init_vel3  eul_0=init_eul3  pm_0=init_ang3  mass_0=M3  mass_e=0.5  mass_f=2.0  inertia=I3  inertia_e=eye(3)  inertia_f=2*eye(3)  k_quat=1.0  vre_flag=on  abi_flag=on  aMode=aMode
      settings: SourceProductBaseCode=AE
  Product : Product  Multiplication=Matrix(*)
  Terminator1 : Terminator
  Terminator2 : Terminator
  Terminator3 : Terminator
  Vector Concatenate{,1..3} (4 alike) : Concatenate
  q1e : Outport
  q1_dote : Outport  Port=2
  q1 : Outport  Port=3
  q1_dotb : Outport  Port=4
  Xe1 : Outport  Port=5
  DCMbe1 : Outport  Port=6
  wires:
  Vector Concatenate2/1 -> q1e/1  "q1"
  Vector Concatenate3/1 -> q1_dote/1  "q1_dot"
  6DOF (Euler Angles) Node 1/7 -> Terminator1/1
  6DOF (Euler Angles) Node 1/6 -> Vector Concatenate3/2, Vector Concatenate1/2
  6DOF (Euler Angles) Node 1/8 -> Terminator2/1
  6DOF (Euler Angles) Node 1/5 -> Vector Concatenate1/1
  Product/1 -> Vector Concatenate/1
  Vector Concatenate1/1 -> q1_dotb/1  "q1_dot"
  6DOF (Euler Angles) Node 1/1 -> Vector Concatenate3/1
  "F_{xyz}"/1 -> 6DOF (Euler Angles) Node 1/1
  6DOF (Euler Angles) Node 1/3 -> Vector Concatenate2/2, Vector Concatenate/2
  "M_{xyz}"/1 -> 6DOF (Euler Angles) Node 1/2
  Vector Concatenate/1 -> q1/1  "q1"
  6DOF (Euler Angles) Node 1/2 -> Xe1/1, Product/2, Vector Concatenate2/1
  6DOF (Euler Angles) Node 1/4 -> DCMbe1/1, Product/1
  6DOF (Euler Angles) Node 1/9 -> Terminator3/1

== system UAV_sync_unknown/Node 3/Subsystem ==
  note: C_Part
  note: theta_C
  note: q1_dotb
  note: -S1.Bm'.P.e.q_dot
  note: -S1.Bm'.P.e.q_dot.Xi_C
  -S1.Bm'.P.e : Inport
  q1_dot_b : Inport  Port=2
  Integrator1 : Integrator
  Product{3..4,6..7} (4 alike) : Product  Multiplication=Matrix(*)
  Reshape3 : Reshape  OutputDimensionality=Row vector (2-D)
  Reshape5 : Reshape  OutputDimensionality=Column vector (2-D)
  To Workspace1 : ToWorkspace  Commented=on  VariableName=Theta_C  SaveFormat=Structure With Time  SampleTime=-1
      settings: Decimation=2
  Transpose1 : Math  Operator=transpose  SaturateOnIntegerOverflow=on
  "Xi_C " : MATLAB Function  TreatAsAtomicUnit=on
  C*q1 : Outport
  wires:
  Product3/1 -> Product4/1
  Transpose1/1 -> Product6/2
  Reshape5/1 -> C*q1/1
  Reshape3/1 -> Product3/2
  -S1.Bm'.P.e/1 -> Product3/1
  Product4/1 -> Integrator1/1
  "Xi_C "/1(y) -> Transpose1/1, Product4/2
  Product6/1 -> Product7/1
  q1_dot_b/1 -> Reshape3/1, Product7/2, "Xi_C "/1(u)
  Product7/1 -> Reshape5/1
  Integrator1/1 -> To Workspace1/1, Product6/1

== system UAV_sync_unknown/Node 3/Subsystem1 ==
  note: D_Part
  note: theta_D
  note: Xi_D=> eye(6)
  note: -S1.Bm'.P.e.()
  (-Kpq-Kvq_dot+r) : Inport
  -S1.Bm'.P.e : Inport  Port=2
  Integrator : Integrator
  Product2 : Product  Multiplication=Matrix(*)
  Product5 : Product  Multiplication=Matrix(*)
  Reshape2 : Reshape  OutputDimensionality=Row vector (2-D)
  Reshape4 : Reshape  OutputDimensionality=Column vector (2-D)
  Reshape6 : Reshape  OutputDimensionality=Column vector (2-D)
  To Workspace : ToWorkspace  Commented=on  VariableName=Theta_D  SaveFormat=Structure With Time  SampleTime=-1
      settings: Decimation=2
  D(-Kpq-Kvq_dot+r) : Outport
  wires:
  Reshape6/1 -> D(-Kpq-Kvq_dot+r)/1
  -S1.Bm'.P.e/1 -> Product2/1
  Reshape4/1 -> Product5/2
  Product2/1 -> Integrator/1
  Integrator/1 -> Product5/1, To Workspace/1
  (-Kpq-Kvq_dot+r)/1 -> Reshape2/1
  Reshape2/1 -> Reshape4/1, Product2/2
  Product5/1 -> Reshape6/1

== system UAV_sync_unknown/Node 3/Subsystem2 ==
  note: -S1.Bm'.P.e
  e : Inport
  Constant : Constant  Value=-100*S1*Bm'
  P : Gain  Gain=Pm  Multiplication=Matrix(u*K)
  Product1 : Product  Multiplication=Matrix(*)
  -S1.Bm'.P.e : Outport
  wires:
  Product1/1 -> -S1.Bm'.P.e/1
  e/1 -> Product1/2
  P/1 -> Product1/1
  Constant/1 -> P/1

== system UAV_sync_unknown/Node 3/Subsystem3 ==
  r : Inport
  q1 : Inport  Port=2
  q1_dot : Inport  Port=3
  Gain1 : Gain  Gain=Kv  Multiplication=Matrix(K*u)
  Gain2 : Gain  Gain=Kp  Multiplication=Matrix(K*u)
  Sum : Sum  Inputs=-+-
  (-Kpq-Kvq_dot+r) : Outport
  wires:
  Sum/1 -> (-Kpq-Kvq_dot+r)/1
  r/1 -> Sum/2
  Gain2/1 -> Sum/1
  q1_dot/1 -> Gain1/1
  Gain1/1 -> Sum/3
  q1/1 -> Gain2/1

== system UAV_sync_unknown/Node 4/Node2_6DOF ==
  "F_{xyz}" : Inport
  "M_{xyz}" : Inport  Port=2
  6DOF (Euler Angles) Node 4 : shared6dof/6DOF (Euler Angles)  units=Metric (MKS)  mtype=Fixed  rep=Euler Angles  xme_0=init_pos4  Vm_0=init_vel4  eul_0=init_eul4  pm_0=init_ang4  mass_0=M4  mass_e=0.5  mass_f=2.0  inertia=I1  inertia_e=eye(3)  inertia_f=2*eye(3)  k_quat=1.0  vre_flag=on  abi_flag=on  aMode=aMode
      settings: SourceProductBaseCode=AE
  Product : Product  Multiplication=Matrix(*)
  Terminator1 : Terminator
  Terminator2 : Terminator
  Terminator3 : Terminator
  Vector Concatenate{,1..3} (4 alike) : Concatenate
  q4e : Outport
  q4_dote : Outport  Port=2
  q4b : Outport  Port=3
  q4_dotb : Outport  Port=4
  Xe4 : Outport  Port=5
  DCMbe4 : Outport  Port=6
  omega_b4 : Outport  Port=7
  wires:
  "M_{xyz}"/1 -> 6DOF (Euler Angles) Node 4/2
  Vector Concatenate1/1 -> q4_dotb/1  "q4_dot"
  "F_{xyz}"/1 -> 6DOF (Euler Angles) Node 4/1
  6DOF (Euler Angles) Node 4/8 -> Terminator2/1
  Vector Concatenate/1 -> q4b/1  "q4"
  6DOF (Euler Angles) Node 4/9 -> Terminator3/1
  Product/1 -> Vector Concatenate/1
  Vector Concatenate2/1 -> q4e/1  "q4"
  Vector Concatenate3/1 -> q4_dote/1  "q4_dot"
  6DOF (Euler Angles) Node 4/7 -> Terminator1/1
  6DOF (Euler Angles) Node 4/1 -> Vector Concatenate3/1
  6DOF (Euler Angles) Node 4/2 -> Vector Concatenate2/1, Xe4/1, Product/2
  6DOF (Euler Angles) Node 4/4 -> DCMbe4/1, Product/1
  6DOF (Euler Angles) Node 4/3 -> Vector Concatenate2/2, Vector Concatenate/2
  6DOF (Euler Angles) Node 4/6 -> Vector Concatenate3/2, omega_b4/1, Vector Concatenate1/2
  6DOF (Euler Angles) Node 4/5 -> Vector Concatenate1/1

== system UAV_sync_unknown/Node 0/Node 0/Derived Data ==
  note: WAE = Wind Angle Error
  In1 : Inport
  In2 : Inport  Port=2
  Bus Creator2 : BusCreator  Inputs=7
  Bus Selector : BusSelector  OutputSignals=WindVelocity(Body)
  Bus Selector5 : BusSelector  OutputSignals=Velocity (body),Velocity (inertial),Euler angles (rad)
  Constant9 : Constant  Value=C_rho
  Dynamic Pressure : aerolibasang/Dynamic Pressure
  "Incidence, Sideslip, & Airspeed" : aerolibasang/Incidence, Sideslip, & Airspeed
      settings: SourceProductName=Aerospace Blockset
  Scope : Scope
  Selector : Selector  InputPortWidth=3  IndexOptions=Index vector (dialog)  Indices=3  OutputSizes=1
  Selector1 : Selector  InputPortWidth=3  IndexOptions=Index vector (dialog)  Indices=2  OutputSizes=1
  Selector3 : Selector  InputPortWidth=3  IndexOptions=Index vector (dialog)  Indices=1  OutputSizes=1
  Sum2 : Sum  Inputs=|-+
  Sum4 : Sum  Inputs=+-|
  Sum5 : Sum  Inputs=+-|
  Trigonometric Function1 : Trigonometry  Operator=atan2
  Derived_Condition : Outport
  wires:
  In2/1 -> Bus Selector5/1
  "Incidence, Sideslip, & Airspeed"/2 -> Sum5/2, Bus Creator2/2  "beta"
  "Incidence, Sideslip, & Airspeed"/1 -> Bus Creator2/1  "alpha"
  Dynamic Pressure/1 -> Bus Creator2/4  "qbar"
  Sum2/1 -> "Incidence, Sideslip, & Airspeed"/1
  Constant9/1 -> Dynamic Pressure/2
  Bus Selector5/2 -> Selector1/1, Selector3/1  "<Velocity (inertial)>"
  Trigonometric Function1/1 -> Sum4/1, Bus Creator2/5  "course_angle"
  Bus Selector5/3 -> Selector/1  "<Euler angles (rad)>"
  Selector/1 -> Sum4/2
  Sum5/1 -> Bus Creator2/7  "WAE"
  "Incidence, Sideslip, & Airspeed"/3 -> Scope/1, Bus Creator2/3  "Va"
  Sum4/1 -> Sum5/1, Bus Creator2/6  "crab_angle"
  Bus Selector5/1 -> Dynamic Pressure/1, Sum2/2  "<Velocity (body)>"
  Bus Creator2/1 -> Derived_Condition/1
  In1/1 -> Bus Selector/1
  Bus Selector/1 -> Sum2/1  "<WindVelocity(Body)>"
  Selector1/1 -> Trigonometric Function1/1
  Selector3/1 -> Trigonometric Function1/2

== system UAV_sync_unknown/Node 0/Node 0/Inverse Dynamics Control ==
  References : Inport
  Aircraft Data : Inport  Port=2
  Constant8 : Constant  Value=g0
  Inverse Dynamic 1 : Subsystem
  Inverse Dynamic 2 : Subsystem
  D_qddot : Outport
  C_qdot : Outport  Port=2
  g(q) : Outport  Port=3
  wires:
  Inverse Dynamic 1/1(D_qddot) -> D_qddot/1
  References/1 -> Inverse Dynamic 1/1(References)
  Aircraft Data/1 -> Inverse Dynamic 2/1(Aricraft Data), Inverse Dynamic 1/2(Aircraft Data)
  Inverse Dynamic 2/1(C_qdot) -> C_qdot/1
  Constant8/1 -> g(q)/1

== system UAV_sync_unknown/Node 0/Node 0/Subsystem ==
  VF_System_Parameters : Inport
  Bus Creator1 : BusCreator  Inputs=18
  Demux : Demux  Outputs=18
  References : Outport
  wires:
  VF_System_Parameters/1 -> Demux/1
  Demux/7 -> Bus Creator1/7  "xdot_ref_final"
  Demux/6 -> Bus Creator1/6  "psi_ref_final"
  Demux/9 -> Bus Creator1/9  "hdot_ref_final"
  Demux/18 -> Bus Creator1/18  "psiddot_ref_final"
  Bus Creator1/1 -> References/1
  Demux/1 -> Bus Creator1/1  "x_ref _final"
  Demux/4 -> Bus Creator1/4  "phi_ref_final"
  Demux/5 -> Bus Creator1/5  "theta_ref_final"
  Demux/2 -> Bus Creator1/2  "y_ref_final"
  Demux/3 -> Bus Creator1/3  "h_ref_final"
  Demux/8 -> Bus Creator1/8  "ydot_ref_final"
  Demux/14 -> Bus Creator1/14  "yddot_ref_final"
  Demux/16 -> Bus Creator1/16  "phiddot_ref_final"
  Demux/15 -> Bus Creator1/15  "hddot_ref_final"
  Demux/10 -> Bus Creator1/10  "phidot_ref_final"
  Demux/13 -> Bus Creator1/13  "xddot_ref_final"
  Demux/17 -> Bus Creator1/17  "thetaddot_ref_final"
  Demux/12 -> Bus Creator1/12  "psidot_ref_final"
  Demux/11 -> Bus Creator1/11  "thetadot_ref_final"

== system UAV_sync_unknown/Node 0/Node 0/Wind ==
  In1 : Inport
  Bus Creator1 : BusCreator  Inputs=1
  Bus Selector4 : BusSelector  OutputSignals=MatrixTransformation(Inertial-Body)
  Constant1 : Constant  Value=InitWind
  Product : Product  Multiplication=Matrix(*)
  Out1 : Outport
  wires:
  Constant1/1 -> Product/2
  In1/1 -> Bus Selector4/1
  Bus Selector4/1 -> Product/1  "<MatrixTransformation(Inertial-Body)>"
  Product/1 -> Bus Creator1/1  "WindVelocity(Body)"
  Bus Creator1/1 -> Out1/1

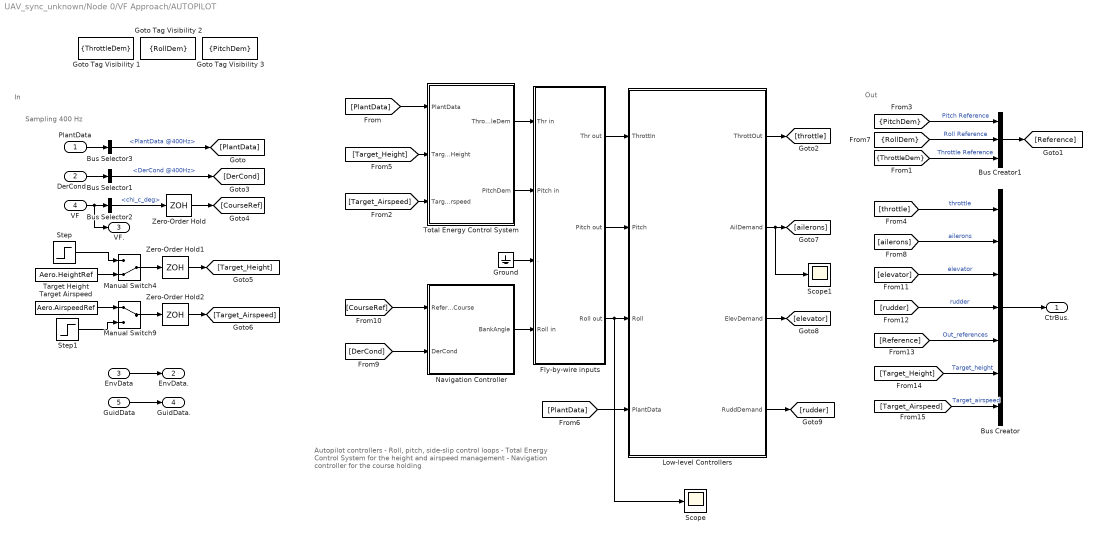
== system UAV_sync_unknown/Node 0/VF Approach/AUTOPILOT ==
  note: In
  note: Out
  note: Autopilot controllers
      |
      | - Roll, pitch, side-slip control loops
      | - Total Energy Control System for the height and airspeed management
      | - Navigation controller for the course holding
  note: Sampling 400 Hz
  PlantData : Inport
  DerCond : Inport  Port=2
  EnvData : Inport  Port=3
  VF : Inport  Port=4
  GuidData : Inport  Port=5
  Bus Creator : BusCreator  Inputs=7
  Bus Creator1 : BusCreator  Inputs=3
  Bus Selector1 : BusSelector  OutputSignals=DerCond @400Hz
  Bus Selector2 : BusSelector  OutputSignals=chi_c_deg
  Bus Selector3 : BusSelector  OutputSignals=PlantData @400Hz
  Fly-by-wire inputs : Subsystem
  Goto Tag Visibility 1 : GotoTagVisibility  GotoTag=ThrottleDem
  Goto Tag Visibility 2 : GotoTagVisibility  GotoTag=RollDem
  Goto Tag Visibility 3 : GotoTagVisibility  GotoTag=PitchDem
  Ground : Ground
  Low-level Controllers : Subsystem
  Manual Switch4 : ManualSwitch  CurrentSetting=0
  Manual Switch9 : ManualSwitch
  Navigation Controller : Subsystem
  Scope : Scope
  Scope1 : Scope
  Step : Step  Time=10  Before=50  After=80  SampleTime=0
  Step1 : Step  Time=10  Before=15  After=20  SampleTime=0
  Target Airspeed : Constant  Value=Aero.AirspeedRef
  Target Height : Constant  Value=Aero.HeightRef
  Total Energy Control System : Subsystem
  Zero-Order Hold : ZeroOrderHold  SampleTime=1/400
  Zero-Order Hold1 : ZeroOrderHold  SampleTime=1/400
  Zero-Order Hold2 : ZeroOrderHold  SampleTime=1/400
  CtrBus. : Outport
  EnvData. : Outport  Port=2
  VF. : Outport  Port=3
  GuidData. : Outport  Port=4
  wires:
  Bus Creator1/1 -> [Reference]
  PlantData/1 -> Bus Selector3/1
  Low-level Controllers/4(RuddDemand) -> [rudder]
  Low-level Controllers/3(ElevDemand) -> [elevator]
  Low-level Controllers/2(AilDemand) -> Scope1/1, [ailerons]
  Low-level Controllers/1(ThrottOut) -> [throttle]
  [RollDem] -> Bus Creator1/2  "Roll Reference"
  [CourseRef] -> Navigation Controller/1(ReferenceCourse)
  [PlantData] -> Low-level Controllers/4(PlantData)
  Bus Selector1/1 -> [DerCond]  "<DerCond @400Hz>"
  DerCond/1 -> Bus Selector1/1
  [DerCond] -> Navigation Controller/2(DerCond)
  Bus Selector3/1 -> [PlantData]  "<PlantData @400Hz>"
  Manual Switch4/1 -> Zero-Order Hold1/1
  Manual Switch9/1 -> Zero-Order Hold2/1
  Step/1 -> Manual Switch4/1
  Target Height/1 -> Manual Switch4/2
  Target Airspeed/1 -> Manual Switch9/1
  Step1/1 -> Manual Switch9/2
  [PitchDem] -> Bus Creator1/1  "Pitch Reference"
  Zero-Order Hold/1 -> [CourseRef]
  [PlantData] -> Total Energy Control System/1(PlantData)
  EnvData/1 -> EnvData./1
  GuidData/1 -> GuidData./1
  VF/1 -> VF./1, Bus Selector2/1
  Bus Selector2/1 -> Zero-Order Hold/1  "<chi_c_deg>"
  [ThrottleDem] -> Bus Creator1/3  "Throttle Reference"
  Zero-Order Hold1/1 -> [Target_Height]
  Zero-Order Hold2/1 -> [Target_Airspeed]
  Total Energy Control System/1(ThrottleDem) -> Fly-by-wire inputs/1(Thr in)
  Total Energy Control System/2(PitchDem) -> Fly-by-wire inputs/2(Pitch in)
  Navigation Controller/1(BankAngle) -> Fly-by-wire inputs/4(Roll in)
  Fly-by-wire inputs/1(Thr out) -> Low-level Controllers/1(ThrottIn)
  Fly-by-wire inputs/2(Pitch out) -> Low-level Controllers/2(Pitch)
  Ground/1 -> Fly-by-wire inputs/3(.)
  [Target_Height] -> Total Energy Control System/2(Target_Height)
  [Target_Airspeed] -> Total Energy Control System/3(Target_Airspeed)
  [ailerons] -> Bus Creator/2  "ailerons"
  [throttle] -> Bus Creator/1  "throttle"
  [elevator] -> Bus Creator/3  "elevator"
  [rudder] -> Bus Creator/4  "rudder"
  [Reference] -> Bus Creator/5  "Out_references"
  [Target_Height] -> Bus Creator/6  "Target_height"
  [Target_Airspeed] -> Bus Creator/7  "Target_airspeed"
  Bus Creator/1 -> CtrBus./1
  Fly-by-wire inputs/3(Roll out) -> Low-level Controllers/3(Roll), Scope/1

== system UAV_sync_unknown/Node 0/VF Approach/BIXLER DYNAMICS ==
  note: This sub-block contains the dynamics of the aircraft.
      |
      | - All the states and quantities of interest are contained in the Bus signal PlantData.
      | - The derived conditions such as Airspeed, Angle of Attack, and Side-slip angle, are contained in Bus signal DerCond .
      | - The Bus EnvData contains the wind quantities of interest.
      | - The dynamical model is continuous, but the Buses are sampled to feed the discrete-time control system.
      | - The parameters of this block are contained in parameters/parameters_aero.
  ControlActions : Inport
  EnvData : Inport  Port=2
  GuidData : Inport  Port=3
  VF : Inport  Port=4
  Actuator Dynamics : Subsystem
  Bus Creator1 : BusCreator  Inputs='qbar','alpha','beta','Va','Course','CrabAngle','WAE'
  Bus Selector : BusSelector  OutputSignals=throttle
  Derived Conditions : Subsystem
  RUBBISH BIN : Subsystem
  Sampling : Subsystem
  "Sampling " : Subsystem
  Throttle Dynamics : Subsystem
  Vehicle Airframe : Subsystem
  PlantData. : Outport
  DerCond. : Outport  Port=2
  ControlBus. : Outport  Port=3
  GuidData. : Outport  Port=4
  VF. : Outport  Port=5
  wires:
  Bus Creator1/1 -> "Sampling "/1(Cont.), [DerCond]  "DerCond"
  Bus Selector/1 -> Throttle Dynamics/1(In)  "<throttle>"
  Throttle Dynamics/1(Out) -> Vehicle Airframe/1(Throttle_cmd)  "throttle"
  ControlActions/1 -> ControlBus./1, Bus Selector/1, Actuator Dynamics/1(In)
  Actuator Dynamics/1(Out) -> Vehicle Airframe/2(ControlActions)
  Vehicle Airframe/1(PlantData) -> [PlantData], Sampling/1(Cont.)  "PlantData"
  Sampling/1(Cont.+Disc.) -> PlantData./1
  "Sampling "/1(Cont.+Disc.) -> DerCond./1
  GuidData/1 -> GuidData./1
  VF/1 -> VF./1
  [PlantData] -> Derived Conditions/2(PlantData)
  EnvData/1 -> Derived Conditions/1(EnvData)
  Derived Conditions/1(qbar) -> Bus Creator1/1  "qbar"
  Derived Conditions/2(alpha) -> Bus Creator1/2  "alpha"
  Derived Conditions/4(Va) -> Bus Creator1/4  "Va"
  Derived Conditions/3(beta) -> Bus Creator1/3  "beta"
  Derived Conditions/5(CourseAngle) -> Bus Creator1/5  "Course"
  Derived Conditions/6(CrabAngle) -> Bus Creator1/6  "CrabAngle"
  Derived Conditions/7(WAE) -> Bus Creator1/7  "WAE"
  [DerCond] -> Vehicle Airframe/3(DerCond)

== system UAV_sync_unknown/Node 0/VF Approach/ENVIRONMENT ==
  note: Wind slowly time varying
  note: Dynamic wind
  note: Constant wind
  PlantData : Inport
  Bus Creator : BusCreator  Inputs=4
  Bus Selector1 : BusSelector  OutputSignals=xyh,Velocity (inertial),From inertial to body matrix
  Bus Selector2 : BusSelector  OutputSignals=From inertial to body matrix
  Bus Selector3 : BusSelector  OutputSignals=PlantData
  Bus Selector4 : BusSelector  OutputSignals=From inertial to body matrix
  Constant1 : Constant  Value=Init.windConst
  Dot Product : DotProduct  InputSameDT=on  OutDataTypeStr=Inherit: Inherit via internal rule
  Dryden Wind Turbulence Model (Continuous (+q +r)) : aerolibwind2/Dryden Wind Turbulence Model  (Continuous (+q -r))  units=Metric (MKS)  spec=MIL-F-8785C  model=Continuous Dryden (+q +r)  W20=10  Wdeg=135  TurbProb=10^-2 - Light  L_high=533.4  Wingspan=Bxl.b  ts=0.1  Seed=[23341 23342 23343 23344]  T_on=on
      settings: SourceProductName=Aerospace Blockset
  Height : Selector  InputPortWidth=3  IndexOptions=Index vector (dialog)  Indices=3  OutputSizes=1
  Init.DryOnOff : Gain  Gain=Init.DryOnOff
  "Init.DryOnOff " : Gain  Gain=Init.DryOnOff
  Init.WTimevar : Gain  Gain=Init.WTimevar
  Product : Product  Multiplication=Matrix(*)
  "Product " : Product  Multiplication=Matrix(*)
  Slowly time varying wind gen. : Subsystem
  Sum1 : Sum  Inputs=|++
  Sum3 : Sum  Inputs=|++
  Vt : Sqrt  SaturateOnIntegerOverflow=on
  EnvData : Outport
  wires:
  Bus Selector1/1 -> Height/1  "<xyh>"
  Bus Selector1/2 -> Dot Product/2, Dot Product/1  "<Velocity (inertial)>"
  Bus Selector1/3 -> Dryden Wind Turbulence Model (Continuous (+q +r))/3  "<From inertial to body matrix>"
  Bus Selector3/1 -> Bus Selector4/1, Bus Selector1/1, Bus Selector2/1  "<PlantData>"
  Height/1 -> Dryden Wind Turbulence Model (Continuous (+q +r))/1  "Altitude"
  Dot Product/1 -> Vt/1
  Vt/1 -> Dryden Wind Turbulence Model (Continuous (+q +r))/2  "Speed"
  Sum1/1 -> Bus Creator/3, Sum3/2  "Wind velocity (dyn) (body)"
  Constant1/1 -> Product/2
  Bus Creator/1 -> EnvData/1
  "Init.DryOnOff "/1 -> Bus Creator/4  "Wind ang rate (dyn) (body)"
  Sum3/1 -> Bus Creator/2  "Wind total (body)"
  Dryden Wind Turbulence Model (Continuous (+q +r))/1 -> Init.DryOnOff/1
  Bus Selector2/1 -> Product/1  "<From inertial to body matrix>"
  Dryden Wind Turbulence Model (Continuous (+q +r))/2 -> "Init.DryOnOff "/1
  PlantData/1 -> Bus Selector3/1
  Product/1 -> Bus Creator/1, Sum3/1  "Wind velocity (sta) (body)"
  Bus Selector4/1 -> "Product "/1  "<From inertial to body matrix>"
  Init.WTimevar/1 -> Sum1/2  "Wind slowly time varying"
  Init.DryOnOff/1 -> Sum1/1
  "Product "/1 -> Init.WTimevar/1
  Slowly time varying wind gen./1(Out1) -> "Product "/2
